simulink model "task3"  (R2018a)
settings: Solver=VariableStepAuto  StartTime=0.0  StopTime=10.0  RelTol=1e-3
libraries: dspsnks4 x1
settings Model: Creator=ASITHA  LastModifiedBy=ASITHA

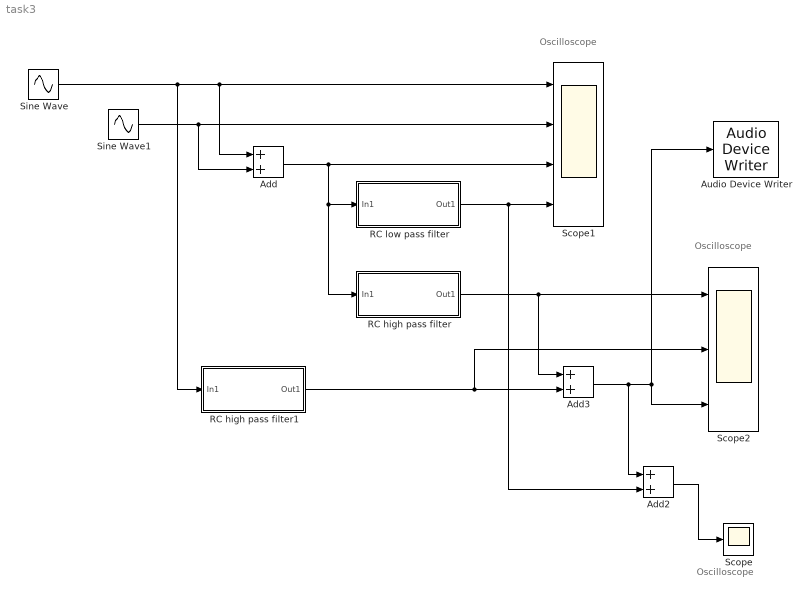
== system task3 ==
  note: Oscilloscope
  note: Oscilloscope
  note: Oscilloscope
  Add : Sum
  Add2 : Sum
  Add3 : Sum
  Audio Device Writer : dspsnks4/Audio Device Writer  Driver=DirectSound  Device=Default  InheritSampleRate=on  SampleRate=44100  BitDepth=16-bit integer  BufferSize=4096  NumBuffers=10  DefaultOutputChannelMapping=on  OutputChannelMapping=1:2  OutputNumUnderrunSamples=off  DriverIdx=1  DeviceWarnFlag=''
  RC high pass filter : Subsystem
  RC high pass filter1 : Subsystem
  RC low pass filter : Subsystem
  Scope : Scope
  Scope1 : Scope  NumInputPorts=4
  Scope2 : Scope  NumInputPorts=3
  Sine Wave : Sin  Amplitude=5  Frequency=1*2*pi  SampleTime=0
  Sine Wave1 : Sin  Amplitude=5  Frequency=5 * 2* pi  SampleTime=0
  wires:
  Sine Wave1/1 -> Add/2, Scope1/2
  Add/1 -> RC high pass filter/1(In1), RC low pass filter/1(In1), Scope1/3
  Sine Wave/1 -> RC high pass filter1/1(In1), Add/1, Scope1/1
  RC high pass filter1/1(Out1) -> Scope2/2, Add3/2
  RC high pass filter/1(Out1) -> Scope2/1, Add3/1
  Add3/1 -> Add2/1, Audio Device Writer/1, Scope2/3
  RC low pass filter/1(Out1) -> Add2/2, Scope1/4
  Add2/1 -> Scope/1

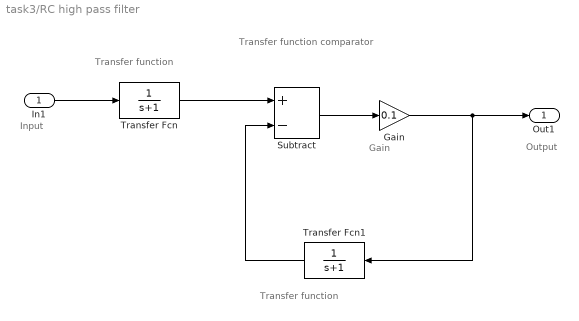
== system task3/RC high pass filter ==
  note: Transfer function
  note: Transfer function
  note: Transfer function comparator
  note: Gain
  note: Input
  note: Output
  In1 : Inport
  Gain : Gain  Gain=0.1
  Subtract : Sum  Inputs=+-
  Transfer Fcn : TransferFcn  Denominator=[1 1]
  Transfer Fcn1 : TransferFcn  Denominator=[1 1]
  Out1 : Outport
  wires:
  In1/1 -> Transfer Fcn/1
  Transfer Fcn/1 -> Subtract/1
  Transfer Fcn1/1 -> Subtract/2
  Gain/1 -> Transfer Fcn1/1, Out1/1
  Subtract/1 -> Gain/1

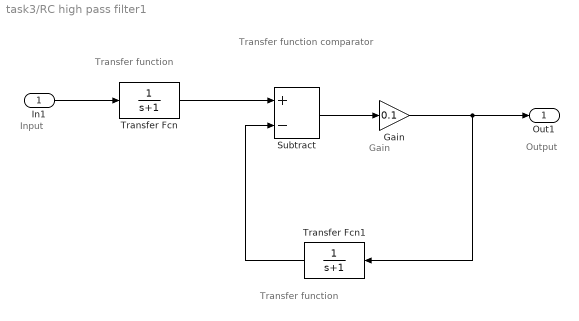
== system task3/RC high pass filter1 ==
  note: Transfer function
  note: Transfer function
  note: Transfer function comparator
  note: Gain
  note: Input
  note: Output
  In1 : Inport
  Gain : Gain  Gain=0.1
  Subtract : Sum  Inputs=+-
  Transfer Fcn : TransferFcn  Denominator=[1 1]
  Transfer Fcn1 : TransferFcn  Denominator=[1 1]
  Out1 : Outport
  wires:
  In1/1 -> Transfer Fcn/1
  Transfer Fcn/1 -> Subtract/1
  Transfer Fcn1/1 -> Subtract/2
  Gain/1 -> Transfer Fcn1/1, Out1/1
  Subtract/1 -> Gain/1

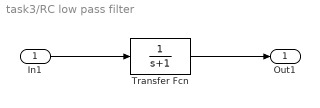
== system task3/RC low pass filter ==
  In1 : Inport
  Transfer Fcn : TransferFcn  Denominator=[1 1]
  Out1 : Outport
  wires:
  In1/1 -> Transfer Fcn/1
  Transfer Fcn/1 -> Out1/1
